simulink model "WirelessChannEfect"  (Simulink 7.7)
settings: Solver=ode45  StartTime=0.0  StopTime=10.0  RelTol=1e-3
undefined symbols (not defined in the file): get
libraries: commsink2 x3, commdigbbndam3 x2, commrandsrc2 x1
settings Model: Creator=horacio  LastModifiedBy=horacio

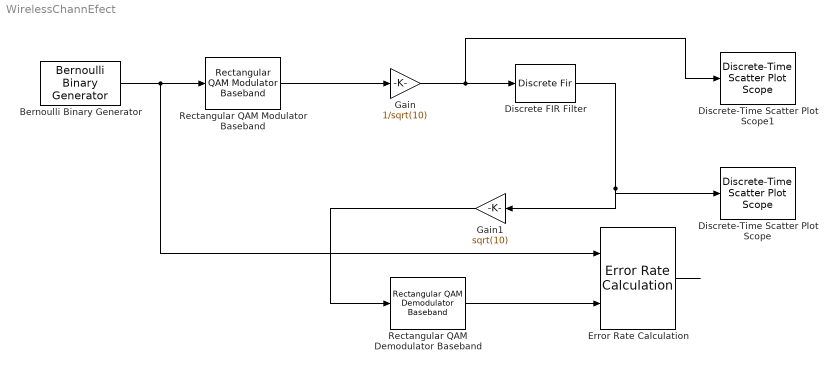
== system WirelessChannEfect ==
  Bernoulli Binary Generator : commrandsrc2/Bernoulli Binary Generator  SystemSampleTime=-1  P=0.5  seed=61  Ts=1/1e6  frameBased=on  sampPerFrame=256  orient=off  outDataType=double
  Discrete FIR Filter : DiscreteFir  NumCoeffs="[1  0  0 0.3 0.1]"  InputProcessing=Columns as channels (frame based)
  Discrete-Time Scatter Plot Scope : commsink2/Discrete-Time Scatter Plot Scope  Tag=ScatterPlot  SystemSampleTime=-1  sampPerSymb=1  offsetEye=0  numTraces=40  numNewFrames=40  LineMarkers=.  LineColors=b  fading=on  render=on  AxisGrid=on  xMin=-3.3  xMax=3.315  yMin=-3.3  yMax=3.315  inphaseLabel=In-phase Amplitude  quadratureLabel=Quadrature Amplitude  openScopeAtSimStart=on  FrameNumber=off  FigPos=get(0,'defaultfigureposition');  figTitle=Scatter Plot  numLinesMax=8  block_type_=scatter
  Discrete-Time Scatter Plot Scope1 : commsink2/Discrete-Time Scatter Plot Scope  Tag=ScatterPlot  SystemSampleTime=-1  sampPerSymb=1  offsetEye=0  numTraces=40  numNewFrames=40  LineMarkers=.  LineColors=b  fading=on  render=on  AxisGrid=on  xMin=-3.3  xMax=3.315  yMin=-3.3  yMax=3.315  inphaseLabel=In-phase Amplitude  quadratureLabel=Quadrature Amplitude  openScopeAtSimStart=on  FrameNumber=off  FigPos=get(0,'defaultfigureposition');  figTitle=Scatter Plot  numLinesMax=8  block_type_=scatter
  Error Rate Calculation : commsink2/Error Rate Calculation  N=0  st_delay=0  cp_mode=Entire frame  subframe=[]  PMode=Port  WsName=ErrorVec  RsMode2=off  stop=off  numErr=100  maxBits=1e6
  Gain : Gain  Gain=1/sqrt(10)
  Gain1 : Gain  Gain=sqrt(10)
  Rectangular QAM Demodulator Baseband : commdigbbndam3/Rectangular QAM Demodulator Baseband  M=2  PowType=Min. distance between symbols  MinDist=2  AvgPow=1  PeakPow=1  Ph=0  Dec=Gray  Mapping=[0:15]  OutType=Bit  DecType=Hard decision  VarSource=Dialog  Variance=1  outDtype1=Inherit via internal rule  outDtype2=Inherit via internal rule  derotateFactorWordLen=16  denormFactorWordLen=16  prodOutWordLen=32  prodOutRoundingMode=Floor  prodOutOverflowMode=Wrap  sumWordLen=32
  Rectangular QAM Modulator Baseband : commdigbbndam3/Rectangular QAM Modulator Baseband  M=2  InType=Bit  Enc=Gray  Mapping=[0:15]  PowType=Min. distance between symbols  MinDist=2  AvgPow=1  PeakPow=1  Ph=0  outDtype=double  outWordLen=16  outUDDataType=sfix(16)  outFracLenMode=Best precision  outFracLen=15
  wires:
  Bernoulli Binary Generator/1 -> Rectangular QAM Modulator Baseband/1, Error Rate Calculation/1
  Rectangular QAM Demodulator Baseband/1 -> Error Rate Calculation/2
  Rectangular QAM Modulator Baseband/1 -> Gain/1
  Gain/1 -> Discrete-Time Scatter Plot Scope1/1, Discrete FIR Filter/1
  Discrete FIR Filter/1 -> Gain1/1, Discrete-Time Scatter Plot Scope/1
  Gain1/1 -> Rectangular QAM Demodulator Baseband/1
  Error Rate Calculation/1 -> ?
